simulink model "DFIPM_LinearModel"  (R2019b)
settings: Solver=FixedStepAuto  StartTime=0.0  StopTime=1  FixedStep=1e-7  RelTol=1e-3
values from neighbouring files (symbols this model uses):
  B = 0.00002    (= 2e-05)    [Parameter_Setting.m]
  duty_limit = 2/sqrt(3)    [Parameter_Setting.m]
  faif = 0.047    [Parameter_Setting.m]
  Iq_limit = 60    [Parameter_Setting.m]
  Jm = 0.00247*2    (= 0.00494)    [Parameter_Setting.m]
  Kawc = Kic/Kpc    (= 106.25)    [Parameter_Setting.m]
  Kic = Rs*wc    (= 106.814150222)    [Parameter_Setting.m]
  Kis = ws^2*Jm/KT    (= 276.628912008)    [Parameter_Setting.m]
  Kpc = Ld*wc    (= 1.00530964915)    [Parameter_Setting.m]
  Kps = yita*ws*2*Jm/KT    (= 3.1126989135)    [Parameter_Setting.m]
  Ld = 0.08e-3    (= 8e-05)    [Parameter_Setting.m]
  Lq = 0.28e-3    (= 0.00028)    [Parameter_Setting.m]
  p = 4    [Parameter_Setting.m]
  Rs = 8.5e-3    (= 0.0085)    [Parameter_Setting.m]
  Ts = 1/(50e3)    (= 2e-05)    [Parameter_Setting.m]
  Ts_spc = Ts    (= 2e-05)    [Parameter_Setting.m]
  VDC = 370    [Parameter_Setting.m]
undefined symbols (not defined in the file or in its folder): DiscIntNeverNeededParam
libraries: simulink x2, powerlib_meascontrol x1, powerlib x1
settings Model: Creator=Downstream  LastModifiedBy=Downstream
settings SolverCC: AlgebraicLoopSolver=LineSearch

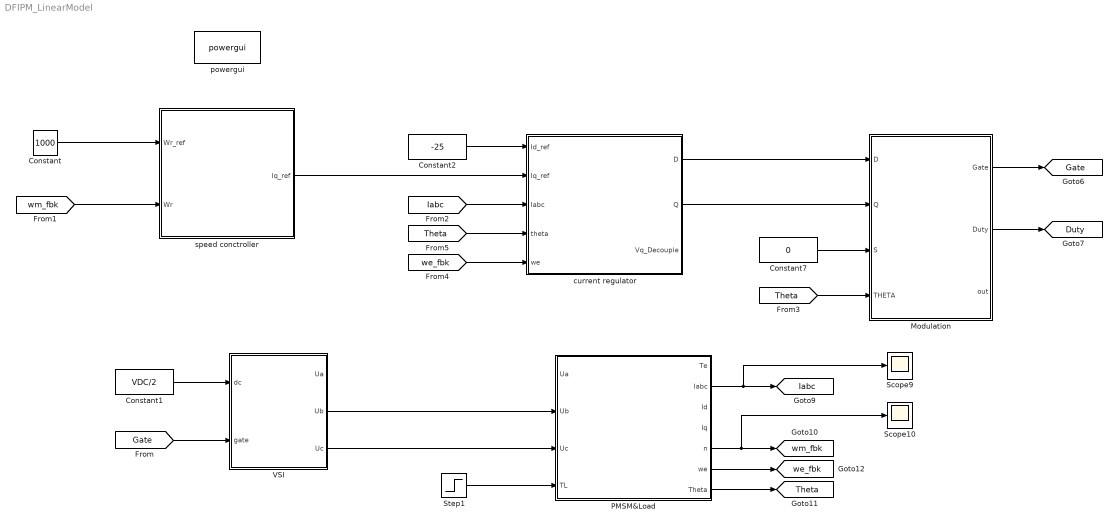
== system DFIPM_LinearModel ==
  Constant : Constant  Value=1000  OutDataTypeStr=Inherit: Inherit via back propagation  SampleTime=-1
  Constant1 : Constant  Value=VDC/2  SampleTime=-1
  Constant2 : Constant  Value=-25  SampleTime=-1
  Constant7 : Constant  Value=0  SampleTime=-1
  Modulation : Subsystem
  "PMSM&Load " : Subsystem
  Scope10 : Scope
  Scope9 : Scope
  Step1 : Step  Time=0.3  After=10
  VSI : Subsystem
  current regulator : Subsystem
  powergui : powerlib/powergui  Priority=1  SimulationMode=Discrete  SampleTime=1e-7  frequency=60  Iterations=50  frequencyindice=60  Pbase=100e6  ErrMax=1e-4  UnitsV=kV  UnitsW=MW  buscounter=0  FunctionMessages=off  echomessages=off  EnableUseOfTLC=off  CurrentSourceSwitches=off  DisableSnubberDevices=off  DisableRonSwitches=off  DisableVfSwitches=off  DisplayEquations=off  AutomaticDiscreteSolvers=off  SolverType=Tustin/Backward Euler (TBE)  Interpol=off  ExternalGateDelay=off  methode=off  Ts=100  x0status=blocks  SPID=on  SwTol=0  HookPort=off  NonlinearTolerance=1e-4  nMaxIteration=100  ContinueOnMaxIteration=off  RestoreLinks=warning  ResistiveCurrentMeasurement=off  Frange=[0:2:500]  Ylog=off  Xlog=on  ShowGrid=off  save=off  variable=ZData  structure=0  ZoomFFT=off  StartTime=0.0  cycles=1  DisplayStyle=1  fundamental=60  FreqAxis=off  MaxFrequency=1000  frequencyindicesteady=1  RmsSteady=1  display=off
      settings: SourceProductName=Simscape Electrical
  speed conctroller : Subsystem
  tag scope: Duty=global, Gate=global, Iabc=global, Theta=global, we_fbk=global, wm_fbk=global
  wires:
  Constant1/1 -> VSI/1(dc)
  VSI/2(Ub) -> "PMSM&Load "/2(Ub)
  VSI/3(Uc) -> "PMSM&Load "/3(Uc)
  [Gate] -> VSI/2(gate)
  speed conctroller/1(Iq_ref) -> current regulator/2(Iq_ref)
  [Iabc] -> current regulator/3(Iabc)
  [Theta] -> current regulator/4(theta)
  [we_fbk] -> current regulator/5(we)
  Modulation/1(Gate) -> [Gate]
  Constant/1 -> speed conctroller/1(Wr_ref)
  [Theta] -> Modulation/4(THETA)
  Constant7/1 -> Modulation/3(S)
  [wm_fbk] -> speed conctroller/2(Wr)
  Constant2/1 -> current regulator/1(Id_ref)
  Modulation/2(Duty) -> [Duty]
  current regulator/1(D) -> Modulation/1(D)
  current regulator/2(Q) -> Modulation/2(Q)
  "PMSM&Load "/2(Iabc) -> Scope9/1, [Iabc]
  "PMSM&Load "/5(n) -> Scope10/1, [wm_fbk]
  "PMSM&Load "/7(Theta) -> [Theta]
  "PMSM&Load "/6(we) -> [we_fbk]
  Step1/1 -> "PMSM&Load "/4(TL)

== system DFIPM_LinearModel/Modulation ==
  D : Inport
  Q : Inport  Port=2
  S : Inport  Port=3
  THETA : Inport  Port=4
  Mux : Mux  Inputs=3
  SVPWM1 : Subsystem
  Zero-Order Hold2 : ZeroOrderHold  SampleTime=Ts
  dq-abcde : Subsystem
  Gate : Outport  VectorParamsAs1DForOutWhenUnconnected=off
  Duty : Outport  Port=2  VectorParamsAs1DForOutWhenUnconnected=off
  out : Outport  Port=3  VectorParamsAs1DForOutWhenUnconnected=off
  wires:
  Q/1 -> dq-abcde/1(q1)
  D/1 -> dq-abcde/2(d1)
  S/1 -> dq-abcde/3(s)
  THETA/1 -> Zero-Order Hold2/1
  dq-abcde/2(B) -> Mux/2
  dq-abcde/3(C) -> Mux/3
  dq-abcde/1(A) -> Mux/1
  Mux/1 -> SVPWM1/1(Duty)
  SVPWM1/1(Gate) -> Gate/1
  Zero-Order Hold2/1 -> dq-abcde/4(Theta)
  SVPWM1/2(DutyCycle) -> Duty/1
  SVPWM1/3(out) -> out/1

== system DFIPM_LinearModel/PMSM&Load  ==
  Ua : Inport
  Ub : Inport  Port=2
  Uc : Inport  Port=3
  TL : Inport  Port=4
  PMSM : Subsystem
  Torque_Producer : Subsystem
  Te : Outport
  Iabc : Outport  Port=2
  Id : Outport  Port=3
  Iq : Outport  Port=4
  n : Outport  Port=5
  we : Outport  Port=6
  Theta : Outport  Port=7
  wires:
  PMSM/1(Te) -> Torque_Producer/2(sigma_Te), Te/1
  PMSM/3(Id) -> Id/1
  Ub/1 -> PMSM/2(Ub)
  Uc/1 -> PMSM/3(Uc)
  PMSM/2(Iabc) -> Iabc/1
  Ua/1 -> PMSM/1(Ua)
  PMSM/4(Iq) -> Iq/1
  TL/1 -> Torque_Producer/1(TL)
  Torque_Producer/1(n) -> n/1
  Torque_Producer/3(theta) -> Theta/1, PMSM/4(Theta)
  Torque_Producer/2(we) -> we/1

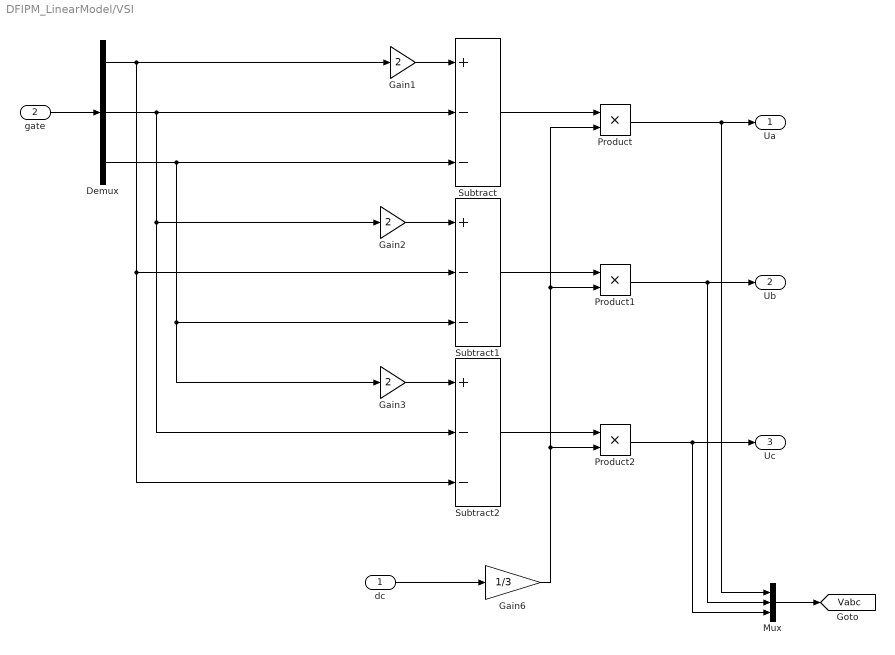
== system DFIPM_LinearModel/VSI ==
  dc : Inport
  gate : Inport  Port=2
  Demux : Demux  Outputs=3
  Gain1 : Gain  Gain=2
  Gain2 : Gain  Gain=2
  Gain3 : Gain  Gain=2
  Gain6 : Gain  Gain=1/3
  Mux : Mux  Inputs=3
  Product : Product  RndMeth=Zero
  Product1 : Product  RndMeth=Zero
  Product2 : Product  RndMeth=Zero
  Subtract : Sum  Inputs=+--
  Subtract1 : Sum  Inputs=+--
  Subtract2 : Sum  Inputs=+--
  Ua : Outport  VectorParamsAs1DForOutWhenUnconnected=off
  Ub : Outport  Port=2  VectorParamsAs1DForOutWhenUnconnected=off
  Uc : Outport  Port=3  VectorParamsAs1DForOutWhenUnconnected=off
  tag scope: Vabc=global
  wires:
  Demux/2 -> Subtract2/2, Gain2/1, Subtract/2
  Demux/3 -> Gain3/1, Subtract1/3, Subtract/3
  Product/1 -> Ua/1, Mux/1
  Product1/1 -> Mux/2, Ub/1
  Product2/1 -> Mux/3, Uc/1
  dc/1 -> Gain6/1
  Demux/1 -> Gain1/1, Subtract1/2, Subtract2/3
  Gain1/1 -> Subtract/1
  Subtract/1 -> Product/1
  Gain6/1 -> Product/2, Product1/2, Product2/2
  Gain2/1 -> Subtract1/1
  Subtract1/1 -> Product1/1
  Gain3/1 -> Subtract2/1
  Subtract2/1 -> Product2/1
  gate/1 -> Demux/1
  Mux/1 -> [Vabc]

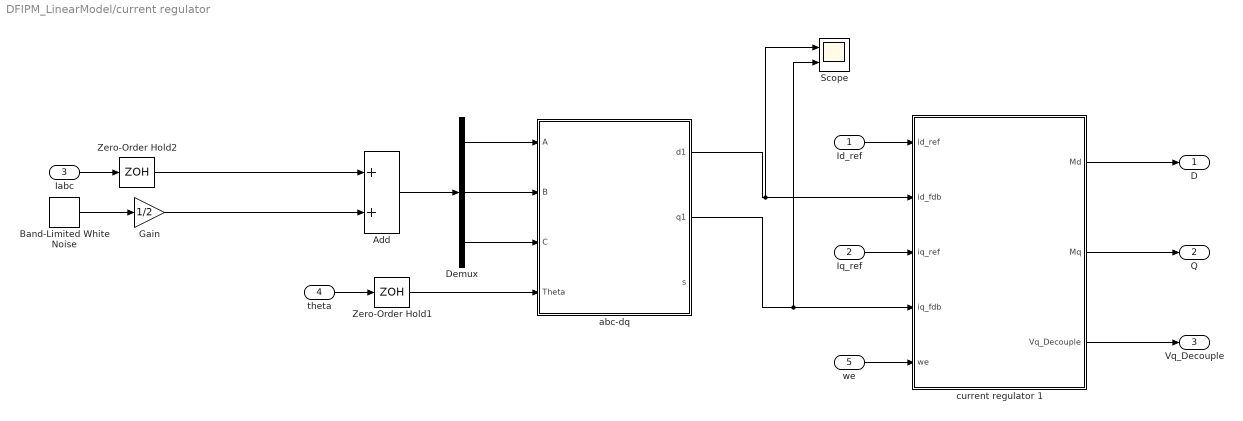
== system DFIPM_LinearModel/current regulator ==
  Id_ref : Inport
  Iq_ref : Inport  Port=2
  Iabc : Inport  Port=3
  theta : Inport  Port=4
  we : Inport  Port=5
  Add : Sum
  Band-Limited White Noise : simulink/Sources/Band-Limited White Noise  Cov=[0.003]  Ts=Ts  seed=[23341]
  Demux : Demux  Outputs=3
  Gain : Gain  Gain=1/2
  Scope : Scope  NumInputPorts=2
  Zero-Order Hold1 : ZeroOrderHold  SampleTime=Ts
  Zero-Order Hold2 : ZeroOrderHold  SampleTime=Ts
  abc-dq : Subsystem
  "current regulator 1 " : Subsystem
  D : Outport  VectorParamsAs1DForOutWhenUnconnected=off
  Q : Outport  Port=2  VectorParamsAs1DForOutWhenUnconnected=off
  Vq_Decouple : Outport  Port=3  VectorParamsAs1DForOutWhenUnconnected=off
  wires:
  Demux/3 -> abc-dq/3(C)
  Demux/1 -> abc-dq/1(A)
  theta/1 -> Zero-Order Hold1/1
  Iabc/1 -> Zero-Order Hold2/1
  Id_ref/1 -> "current regulator 1 "/1(id_ref)
  we/1 -> "current regulator 1 "/5(we)
  "current regulator 1 "/1(Md) -> D/1
  "current regulator 1 "/2(Mq) -> Q/1
  Demux/2 -> abc-dq/2(B)
  Zero-Order Hold1/1 -> abc-dq/4(Theta)
  "current regulator 1 "/3(Vq_Decouple) -> Vq_Decouple/1
  Iq_ref/1 -> "current regulator 1 "/3(iq_ref)
  Band-Limited White Noise/1 -> Gain/1
  Gain/1 -> Add/2
  Zero-Order Hold2/1 -> Add/1
  Add/1 -> Demux/1
  abc-dq/1(d1) -> "current regulator 1 "/2(id_fdb), Scope/1
  abc-dq/2(q1) -> Scope/2, "current regulator 1 "/4(iq_fdb)

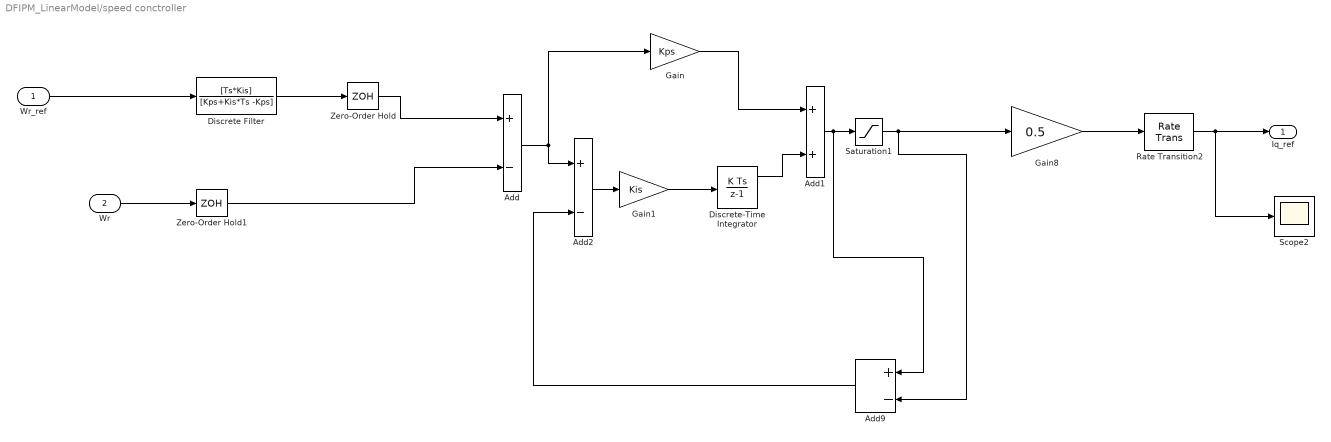
== system DFIPM_LinearModel/speed conctroller ==
  Wr_ref : Inport
  Wr : Inport  Port=2
  Add : Sum  Inputs=+-
  Add1 : Sum
  Add2 : Sum  Inputs=+-
  Add9 : Sum  Inputs=+-
  Discrete Filter : DiscreteFilter  Numerator=[Ts*Kis]  Denominator=[Kps+Kis*Ts -Kps]  SampleTime=Ts
  Discrete-Time Integrator : DiscreteIntegrator  gainval=1  SampleTime=Ts_spc  LimitOutput=on  UpperSaturationLimit=Iq_limit  LowerSaturationLimit=0  ShowSaturationPort=on  ICPrevOutput=DiscIntNeverNeededParam  ICPrevScaledInput=DiscIntNeverNeededParam
  Gain : Gain  Gain=Kps
  Gain1 : Gain  Gain=Kis
  Gain8 : Gain  Gain=0.5
  Rate Transition2 : RateTransition
  Saturation1 : Saturate  UpperLimit=Iq_limit  LowerLimit=-Iq_limit
  Scope2 : Scope
  Zero-Order Hold : ZeroOrderHold  SampleTime=Ts_spc
  Zero-Order Hold1 : ZeroOrderHold  SampleTime=Ts_spc
  Iq_ref : Outport  VectorParamsAs1DForOutWhenUnconnected=off
  wires:
  Gain/1 -> Add1/1
  Wr/1 -> Zero-Order Hold1/1
  Wr_ref/1 -> Discrete Filter/1
  Add1/1 -> Saturation1/1, Add9/1
  Saturation1/1 -> Gain8/1, Add9/2
  Rate Transition2/1 -> Scope2/1, Iq_ref/1
  Zero-Order Hold/1 -> Add/1
  Discrete Filter/1 -> Zero-Order Hold/1
  Discrete-Time Integrator/1 -> Add1/2
  Add/1 -> Add2/1, Gain/1
  Add2/1 -> Gain1/1
  Gain1/1 -> Discrete-Time Integrator/1
  Gain8/1 -> Rate Transition2/1
  Add9/1 -> Add2/2
  Zero-Order Hold1/1 -> Add/2

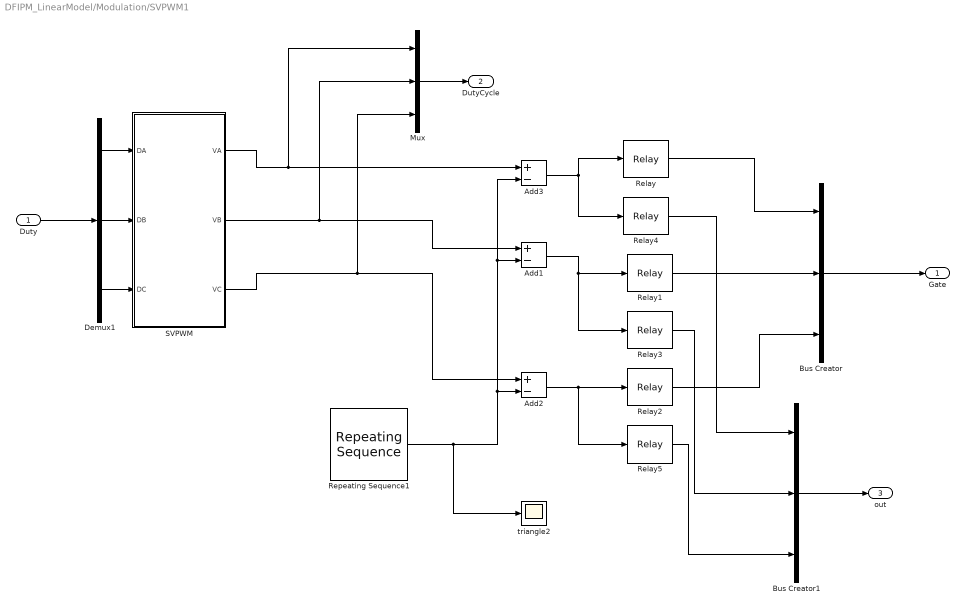
== system DFIPM_LinearModel/Modulation/SVPWM1 ==
  Duty : Inport
  Add1 : Sum  Inputs=+-
  Add2 : Sum  Inputs=+-
  Add3 : Sum  Inputs=+-
  Bus Creator : BusCreator  Inputs=3
  Bus Creator1 : BusCreator  Inputs=3
  Demux1 : Demux  Outputs=3
  Mux : Mux  Inputs=3
  Relay : Relay  OnSwitchValue=0  OffSwitchValue=0  OffOutputValue=-1
  Relay1 : Relay  OnSwitchValue=0  OffSwitchValue=0  OffOutputValue=-1
  Relay2 : Relay  OnSwitchValue=0  OffSwitchValue=0  OffOutputValue=-1
  Relay3 : Relay  OnSwitchValue=0  OffSwitchValue=0
  Relay4 : Relay  OnSwitchValue=0  OffSwitchValue=0
  Relay5 : Relay  OnSwitchValue=0  OffSwitchValue=0
  Repeating Sequence1 : simulink/Sources/Repeating Sequence  rep_seq_t=[0 Ts/2 Ts]  rep_seq_y=[-1 1 -1]
  SVPWM : Subsystem
  triangle2 : Scope
  Gate : Outport  VectorParamsAs1DForOutWhenUnconnected=off
  DutyCycle : Outport  Port=2  VectorParamsAs1DForOutWhenUnconnected=off
  out : Outport  Port=3  VectorParamsAs1DForOutWhenUnconnected=off
  wires:
  Duty/1 -> Demux1/1
  Add3/1 -> Relay/1, Relay4/1
  Add1/1 -> Relay3/1, Relay1/1
  Relay1/1 -> Bus Creator/2
  Add2/1 -> Relay5/1, Relay2/1
  Relay2/1 -> Bus Creator/3
  Relay/1 -> Bus Creator/1
  Bus Creator/1 -> Gate/1
  Demux1/1 -> SVPWM/1(DA)
  Demux1/2 -> SVPWM/2(DB)
  Demux1/3 -> SVPWM/3(DC)
  SVPWM/2(VB) -> Mux/2, Add1/1
  SVPWM/3(VC) -> Mux/3, Add2/1
  SVPWM/1(VA) -> Mux/1, Add3/1
  Mux/1 -> DutyCycle/1
  Repeating Sequence1/1 -> triangle2/1, Add1/2, Add3/2, Add2/2
  Relay4/1 -> Bus Creator1/1
  Relay3/1 -> Bus Creator1/2
  Relay5/1 -> Bus Creator1/3
  Bus Creator1/1 -> out/1

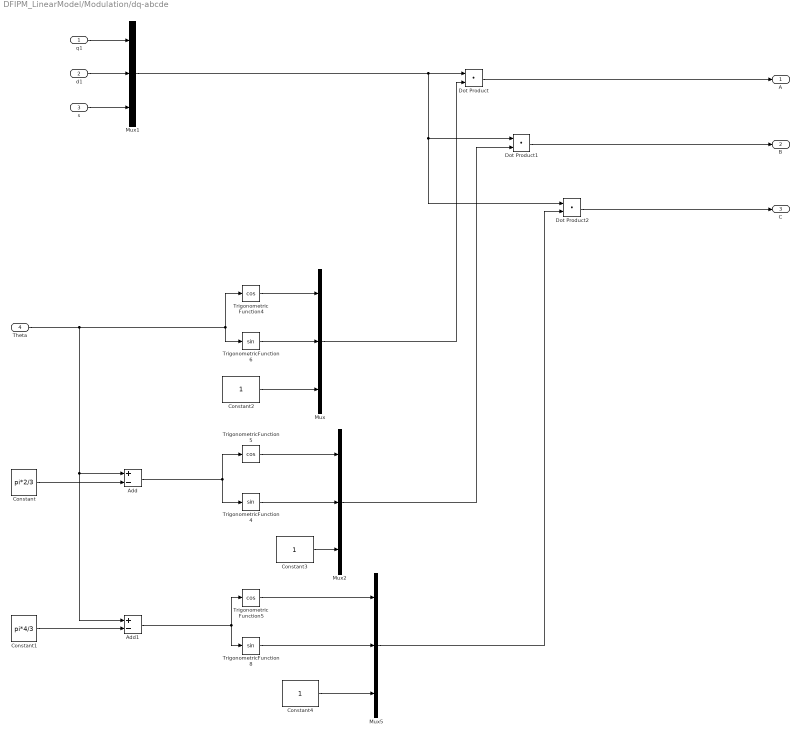
== system DFIPM_LinearModel/Modulation/dq-abcde ==
  q1 : Inport
  d1 : Inport  Port=2
  s : Inport  Port=3
  Theta : Inport  Port=4
  Add : Sum  Inputs=+-
  Add1 : Sum  Inputs=+-
  Constant : Constant  Value=pi*2/3
  Constant1 : Constant  Value=pi*4/3
  Constant2 : Constant
  Constant3 : Constant
  Constant4 : Constant
  Dot Product : DotProduct  InputSameDT=on  OutDataTypeStr=Inherit: Inherit via internal rule
  Dot Product1 : DotProduct  InputSameDT=on  OutDataTypeStr=Inherit: Inherit via internal rule
  Dot Product2 : DotProduct  InputSameDT=on  OutDataTypeStr=Inherit: Inherit via internal rule
  Mux{,1..2,5} (4 alike) : Mux  Inputs=3
  Trigonometric Function4 : Trigonometry  Operator=cos
  Trigonometric Function5 : Trigonometry  Operator=cos
  TrigonometricFunction4 : Trigonometry
  TrigonometricFunction5 : Trigonometry  Operator=cos
  TrigonometricFunction6 : Trigonometry
  TrigonometricFunction8 : Trigonometry
  A : Outport  VectorParamsAs1DForOutWhenUnconnected=off
  B : Outport  Port=2  VectorParamsAs1DForOutWhenUnconnected=off
  C : Outport  Port=3  VectorParamsAs1DForOutWhenUnconnected=off
  wires:
  Theta/1 -> Add/1, Add1/1, Trigonometric Function4/1, TrigonometricFunction6/1
  Constant/1 -> Add/2
  Constant1/1 -> Add1/2
  Add/1 -> TrigonometricFunction5/1, TrigonometricFunction4/1
  Add1/1 -> Trigonometric Function5/1, TrigonometricFunction8/1
  q1/1 -> Mux1/1
  d1/1 -> Mux1/2
  Mux/1 -> Dot Product/2
  Mux1/1 -> Dot Product/1, Dot Product1/1, Dot Product2/1
  Mux2/1 -> Dot Product1/2
  Mux5/1 -> Dot Product2/2
  Trigonometric Function4/1 -> Mux/1
  TrigonometricFunction6/1 -> Mux/2
  TrigonometricFunction5/1 -> Mux2/1
  TrigonometricFunction4/1 -> Mux2/2
  TrigonometricFunction8/1 -> Mux5/2
  Trigonometric Function5/1 -> Mux5/1
  ? -> ?
  Dot Product/1 -> A/1
  Dot Product1/1 -> B/1
  Dot Product2/1 -> C/1
  Constant3/1 -> Mux2/3
  Constant4/1 -> Mux5/3
  Constant2/1 -> Mux/3
  s/1 -> Mux1/3

== system DFIPM_LinearModel/PMSM&Load /PMSM ==
  Ua : Inport
  Ub : Inport  Port=2
  Uc : Inport  Port=3
  Theta : Inport  Port=4
  Mux : Mux  Inputs=3
  Voltage to Current : Subsystem
  abc-dq : Subsystem
  dq-abc : Subsystem
  Te : Outport  VectorParamsAs1DForOutWhenUnconnected=off
  Iabc : Outport  Port=2  VectorParamsAs1DForOutWhenUnconnected=off
  Id : Outport  Port=3  VectorParamsAs1DForOutWhenUnconnected=off
  Iq : Outport  Port=4  VectorParamsAs1DForOutWhenUnconnected=off
  wires:
  abc-dq/2(q1) -> Voltage to Current/2(Uq)
  Mux/1 -> Iabc/1
  dq-abc/3(C) -> Mux/3
  Voltage to Current/3(Te) -> Te/1
  dq-abc/2(B) -> Mux/2
  Voltage to Current/1(Id) -> Id/1, dq-abc/1(d1)
  Ua/1 -> abc-dq/1(A)
  Uc/1 -> abc-dq/3(C)
  Voltage to Current/2(Iq) -> Iq/1, dq-abc/2(q1)
  Ub/1 -> abc-dq/2(B)
  dq-abc/1(A) -> Mux/1
  abc-dq/1(01) -> Voltage to Current/1(Ud)
  Theta/1 -> dq-abc/4(Theta), abc-dq/4(Theta)

== system DFIPM_LinearModel/PMSM&Load /Torque_Producer ==
  TL : Inport
  sigma_Te : Inport  Port=2
  Add4 : Sum  Inputs=+--
  Gain11 : Gain  Gain=B
  Gain12 : Gain  Gain=1/Jm
  Gain13 : Gain  Gain=p
  Gain14 : Gain  Gain=30/pi
  Integrator2 : Integrator
  Integrator3 : Integrator
  n : Outport  VectorParamsAs1DForOutWhenUnconnected=off
  we : Outport  Port=2  VectorParamsAs1DForOutWhenUnconnected=off
  theta : Outport  Port=3  VectorParamsAs1DForOutWhenUnconnected=off
  tag scope: w=global
  wires:
  sigma_Te/1 -> Add4/1
  TL/1 -> Add4/2
  [w] -> Gain11/1
  Gain11/1 -> Add4/3
  Add4/1 -> Gain12/1
  Gain12/1 -> Integrator2/1
  Integrator2/1 -> Gain14/1, [w]
  Integrator3/1 -> theta/1
  [w] -> Gain13/1
  Gain13/1 -> we/1, Integrator3/1
  Gain14/1 -> n/1

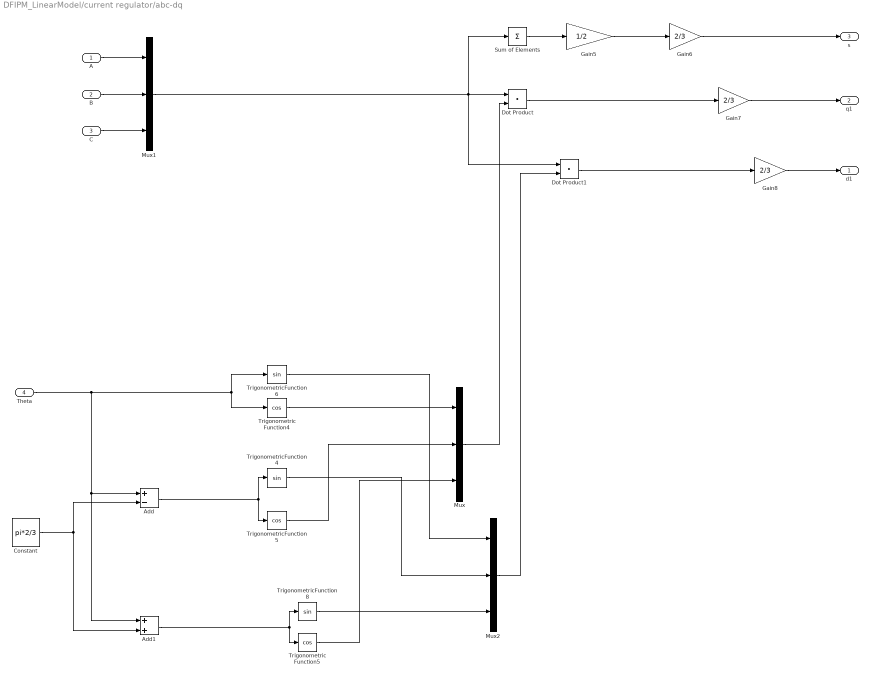
== system DFIPM_LinearModel/current regulator/abc-dq ==
  A : Inport
  B : Inport  Port=2
  C : Inport  Port=3
  Theta : Inport  Port=4
  Add : Sum  Inputs=+-
  Add1 : Sum
  Constant : Constant  Value=pi*2/3
  Dot Product : DotProduct  InputSameDT=on  OutDataTypeStr=Inherit: Inherit via internal rule
  Dot Product1 : DotProduct  InputSameDT=on  OutDataTypeStr=Inherit: Inherit via internal rule
  Gain5 : Gain  Gain=1/2
  Gain6 : Gain  Gain=2/3
  Gain7 : Gain  Gain=2/3
  Gain8 : Gain  Gain=2/3
  Mux : Mux  Inputs=3
  Mux1 : Mux  Inputs=3
  Mux2 : Mux  Inputs=3
  Sum of Elements : Sum  Inputs=+
  Trigonometric Function4 : Trigonometry  Operator=cos
  Trigonometric Function5 : Trigonometry  Operator=cos
  TrigonometricFunction4 : Trigonometry
  TrigonometricFunction5 : Trigonometry  Operator=cos
  TrigonometricFunction6 : Trigonometry
  TrigonometricFunction8 : Trigonometry
  d1 : Outport  VectorParamsAs1DForOutWhenUnconnected=off
  q1 : Outport  Port=2  VectorParamsAs1DForOutWhenUnconnected=off
  s : Outport  Port=3  VectorParamsAs1DForOutWhenUnconnected=off
  wires:
  Theta/1 -> Add/1, Add1/1, TrigonometricFunction6/1, Trigonometric Function4/1
  Constant/1 -> Add/2, Add1/2
  Add/1 -> TrigonometricFunction4/1, TrigonometricFunction5/1
  Add1/1 -> TrigonometricFunction8/1, Trigonometric Function5/1
  A/1 -> Mux1/1
  B/1 -> Mux1/2
  C/1 -> Mux1/3
  Mux/1 -> Dot Product/2
  Mux1/1 -> Dot Product/1, Sum of Elements/1, Dot Product1/1
  Dot Product/1 -> Gain7/1
  Mux2/1 -> Dot Product1/2
  Dot Product1/1 -> Gain8/1
  Sum of Elements/1 -> Gain5/1
  Gain5/1 -> Gain6/1
  Gain6/1 -> s/1
  Gain7/1 -> q1/1
  Gain8/1 -> d1/1
  Trigonometric Function4/1 -> Mux/1
  TrigonometricFunction5/1 -> Mux/2
  Trigonometric Function5/1 -> Mux/3
  TrigonometricFunction6/1 -> Mux2/1
  TrigonometricFunction4/1 -> Mux2/2
  TrigonometricFunction8/1 -> Mux2/3

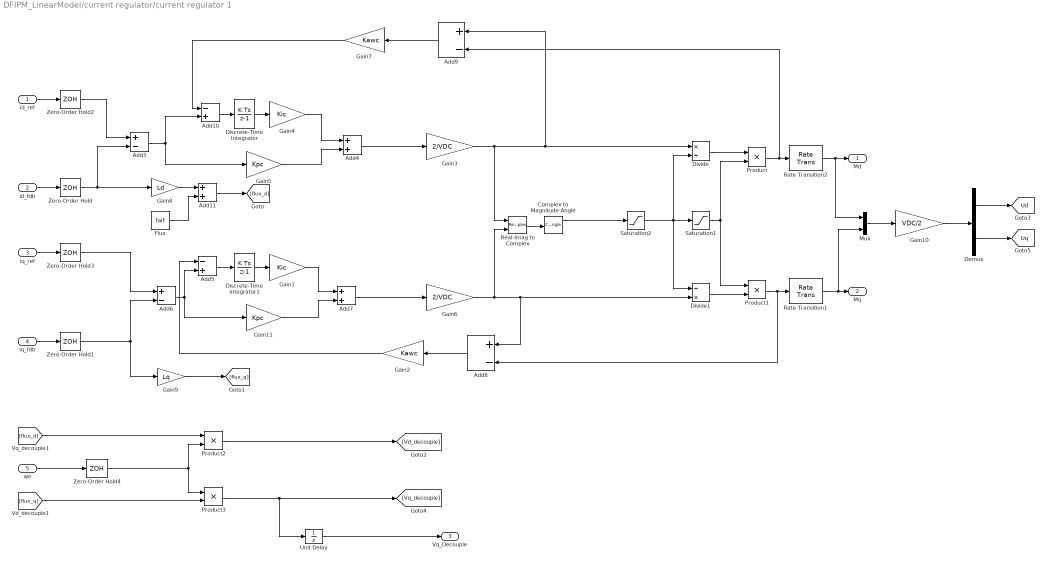
== system DFIPM_LinearModel/current regulator/current regulator 1  ==
  id_ref : Inport
  id_fdb : Inport  Port=2
  iq_ref : Inport  Port=3
  iq_fdb : Inport  Port=4
  we : Inport  Port=5
  Add10 : Sum  Inputs=-+
  Add11 : Sum
  Add{3,6,8..9} (4 alike) : Sum  Inputs=+-
  Add4 : Sum
  Add5 : Sum  Inputs=-+
  Add7 : Sum
  Complex to Magnitude-Angle : ComplexToMagnitudeAngle
  Demux : Demux  Outputs=2
  Discrete-Time Integrator : DiscreteIntegrator  SampleTime=Ts  ICPrevOutput=DiscIntNeverNeededParam  ICPrevScaledInput=DiscIntNeverNeededParam
  Discrete-Time Integrator1 : DiscreteIntegrator  SampleTime=Ts  ICPrevOutput=DiscIntNeverNeededParam  ICPrevScaledInput=DiscIntNeverNeededParam
  Divide : Product  Inputs=*/
  Divide1 : Product  Inputs=/*
  Flux : Constant  Value=faif  SampleTime=-1
  Gain1 : Gain  Gain=Kic
  Gain10 : Gain  Gain=VDC/2
  Gain11 : Gain  Gain=Kpc
  Gain2 : Gain  Gain=Kawc
  Gain3 : Gain  Gain=2/VDC
  Gain4 : Gain  Gain=Kic
  Gain5 : Gain  Gain=Kpc
  Gain6 : Gain  Gain=2/VDC
  Gain7 : Gain  Gain=Kawc
  Gain8 : Gain  Gain=Ld
  Gain9 : Gain  Gain=Lq
  Mux : Mux  Inputs=2
  Product{,1..3} (4 alike) : Product
  Rate Transition1 : RateTransition
  Rate Transition2 : RateTransition
  Real-Imag to Complex : RealImagToComplex
  Saturation1 : Saturate  UpperLimit=duty_limit  LowerLimit=0
  Saturation2 : Saturate  UpperLimit=800  LowerLimit=1e-9
  Unit Delay : UnitDelay  SampleTime=-1  HasFrameUpgradeWarning=on
  Zero-Order Hold{,1..4} (5 alike) : ZeroOrderHold  SampleTime=Ts
  Md : Outport  VectorParamsAs1DForOutWhenUnconnected=off
  Mq : Outport  Port=2  VectorParamsAs1DForOutWhenUnconnected=off
  Vq_Decouple : Outport  Port=3  VectorParamsAs1DForOutWhenUnconnected=off
  tag scope: Ud=global, Uq=global
  wires:
  id_fdb/1 -> Zero-Order Hold/1
  id_ref/1 -> Zero-Order Hold2/1
  Discrete-Time Integrator/1 -> Gain4/1
  Gain4/1 -> Add4/1
  Gain5/1 -> Add4/2
  Zero-Order Hold2/1 -> Add3/1
  Rate Transition2/1 -> Mux/1, Md/1
  Zero-Order Hold/1 -> Gain8/1, Add3/2
  Add3/1 -> Gain5/1, Add10/2
  iq_fdb/1 -> Zero-Order Hold1/1
  iq_ref/1 -> Zero-Order Hold3/1
  Discrete-Time Integrator1/1 -> Gain1/1
  Add6/1 -> Gain11/1, Add5/2
  Gain1/1 -> Add7/1
  Gain11/1 -> Add7/2
  Zero-Order Hold3/1 -> Add6/1
  Zero-Order Hold1/1 -> Gain9/1, Add6/2
  Add5/1 -> Discrete-Time Integrator1/1
  Add4/1 -> Gain3/1
  Add7/1 -> Gain6/1
  Gain3/1 -> Real-Imag to Complex/1, Add9/1, Divide/1
  Real-Imag to Complex/1 -> Complex to Magnitude-Angle/1
  Complex to Magnitude-Angle/1 -> Saturation2/1
  Divide/1 -> Product/1
  Saturation1/1 -> Product/2, Product1/1
  Product/1 -> Add9/2, Rate Transition2/1
  Rate Transition1/1 -> Mux/2, Mq/1
  Gain6/1 -> Real-Imag to Complex/2, Add8/1, Divide1/2
  Product1/1 -> Add8/2, Rate Transition1/1
  Divide1/1 -> Product1/2
  Add8/1 -> Gain2/1
  Gain8/1 -> Add11/1
  Flux/1 -> Add11/2
  Add11/1 -> [flux_d]
  Gain9/1 -> [flux_q]
  [flux_d] -> Product2/1
  we/1 -> Zero-Order Hold4/1
  [flux_q] -> Product3/2
  Product2/1 -> [Vd_decouple]
  Product3/1 -> Unit Delay/1, [Vq_decouple]
  Zero-Order Hold4/1 -> Product3/1, Product2/2
  Gain2/1 -> Add5/1
  Add9/1 -> Gain7/1
  Add10/1 -> Discrete-Time Integrator/1
  Gain7/1 -> Add10/1
  Unit Delay/1 -> Vq_Decouple/1
  Mux/1 -> Gain10/1
  Gain10/1 -> Demux/1
  Demux/1 -> [Ud]
  Demux/2 -> [Uq]
  Saturation2/1 -> Divide1/1, Divide/2, Saturation1/1

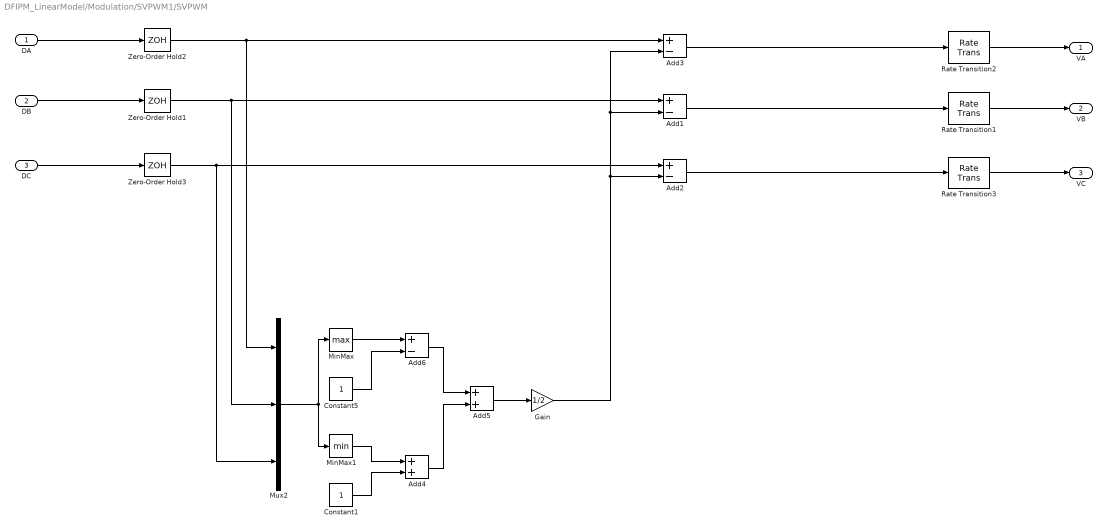
== system DFIPM_LinearModel/Modulation/SVPWM1/SVPWM ==
  DA : Inport
  DB : Inport  Port=2
  DC : Inport  Port=3
  Add{1..3,6} (4 alike) : Sum  Inputs=+-
  Add4 : Sum
  Add5 : Sum
  Constant1 : Constant
  Constant5 : Constant
  Gain : Gain  Gain=1/2
  MinMax : MinMax  Function=max
  MinMax1 : MinMax
  Mux2 : Mux  Inputs=3
  Rate Transition1 : RateTransition  OutPortSampleTime=Ts
  Rate Transition2 : RateTransition  OutPortSampleTime=Ts
  Rate Transition3 : RateTransition  OutPortSampleTime=Ts
  Zero-Order Hold1 : ZeroOrderHold  SampleTime=Ts
  Zero-Order Hold2 : ZeroOrderHold  SampleTime=Ts
  Zero-Order Hold3 : ZeroOrderHold  SampleTime=Ts
  VA : Outport  VectorParamsAs1DForOutWhenUnconnected=off
  VB : Outport  Port=2  VectorParamsAs1DForOutWhenUnconnected=off
  VC : Outport  Port=3  VectorParamsAs1DForOutWhenUnconnected=off
  wires:
  DA/1 -> Zero-Order Hold2/1
  DB/1 -> Zero-Order Hold1/1
  DC/1 -> Zero-Order Hold3/1
  Add2/1 -> Rate Transition3/1
  Add1/1 -> Rate Transition1/1
  Add3/1 -> Rate Transition2/1
  Mux2/1 -> MinMax/1, MinMax1/1
  MinMax/1 -> Add6/1
  Constant5/1 -> Add6/2
  Rate Transition2/1 -> VA/1
  Rate Transition1/1 -> VB/1
  Rate Transition3/1 -> VC/1
  MinMax1/1 -> Add4/1
  Constant1/1 -> Add4/2
  Add6/1 -> Add5/1
  Add4/1 -> Add5/2
  Add5/1 -> Gain/1
  Gain/1 -> Add3/2, Add1/2, Add2/2
  Zero-Order Hold2/1 -> Add3/1, Mux2/1
  Zero-Order Hold1/1 -> Add1/1, Mux2/2
  Zero-Order Hold3/1 -> Add2/1, Mux2/3

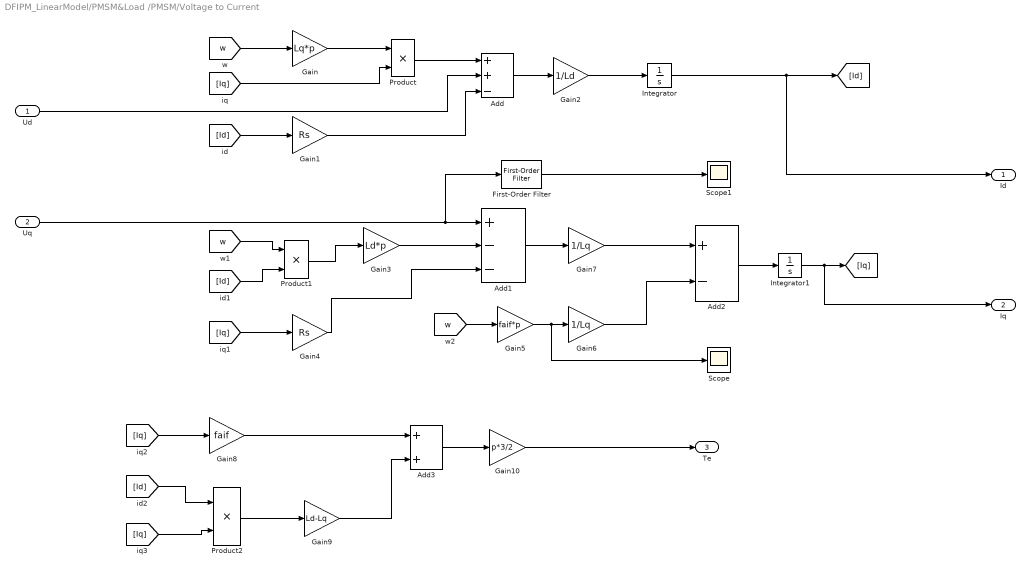
== system DFIPM_LinearModel/PMSM&Load /PMSM/Voltage to Current ==
  Ud : Inport
  Uq : Inport  Port=2
  Add : Sum  Inputs=++-
  Add1 : Sum  Inputs=+--
  Add2 : Sum  Inputs=+-
  Add3 : Sum
  First-Order Filter : powerlib_meascontrol/Filters/First-Order Filter  FilterType=Lowpass  Tc=10e-3  Ts=0  Initialize=off  Vac_Init=[0, 0, 60]  Vdc_Init=0  PlotResponse=off  FreqRange="[0,  200,  1]"
      settings: SourceProductName=Simscape Electrical
  Gain : Gain  Gain=Lq*p
  Gain1 : Gain  Gain=Rs
  Gain10 : Gain  Gain=p*3/2
  Gain2 : Gain  Gain=1/Ld
  Gain3 : Gain  Gain=Ld*p
  Gain4 : Gain  Gain=Rs
  Gain5 : Gain  Gain=faif*p
  Gain6 : Gain  Gain=1/Lq
  Gain7 : Gain  Gain=1/Lq
  Gain8 : Gain  Gain=faif
  Gain9 : Gain  Gain=Ld-Lq
  Integrator : Integrator
  Integrator1 : Integrator
  Product : Product
  Product1 : Product
  Product2 : Product
  Scope : Scope
  Scope1 : Scope
  Id : Outport  VectorParamsAs1DForOutWhenUnconnected=off
  Iq : Outport  Port=2  VectorParamsAs1DForOutWhenUnconnected=off
  Te : Outport  Port=3  VectorParamsAs1DForOutWhenUnconnected=off
  wires:
  Gain/1 -> Product/1
  [Iq] -> Product/2
  [w] -> Gain/1
  Ud/1 -> Add/2
  Product/1 -> Add/1
  [Id] -> Gain1/1
  Gain1/1 -> Add/3
  Add/1 -> Gain2/1
  Uq/1 -> First-Order Filter/1, Add1/1
  [w] -> Product1/1
  [Id] -> Product1/2
  Product1/1 -> Gain3/1
  Gain3/1 -> Add1/2
  [Iq] -> Gain4/1
  Gain4/1 -> Add1/3
  [w] -> Gain5/1
  Gain5/1 -> Scope/1, Gain6/1
  Add1/1 -> Gain7/1
  Gain7/1 -> Add2/1
  Gain6/1 -> Add2/2
  Gain2/1 -> Integrator/1
  Integrator/1 -> Id/1, [Id]
  Add2/1 -> Integrator1/1
  Integrator1/1 -> Iq/1, [Iq]
  [Iq] -> Gain8/1
  Gain8/1 -> Add3/1
  [Id] -> Product2/1
  [Iq] -> Product2/2
  Product2/1 -> Gain9/1
  Gain9/1 -> Add3/2
  Add3/1 -> Gain10/1
  Gain10/1 -> Te/1
  First-Order Filter/1 -> Scope1/1

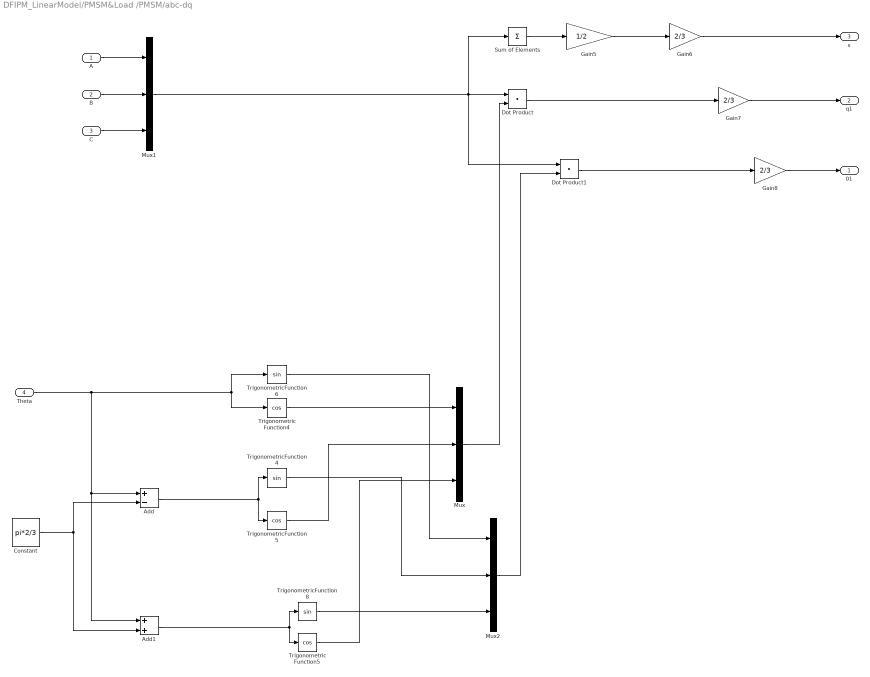
== system DFIPM_LinearModel/PMSM&Load /PMSM/abc-dq ==
  A : Inport
  B : Inport  Port=2
  C : Inport  Port=3
  Theta : Inport  Port=4
  Add : Sum  Inputs=+-
  Add1 : Sum
  Constant : Constant  Value=pi*2/3  SampleTime=-1
  Dot Product : DotProduct  InputSameDT=on  OutDataTypeStr=Inherit: Inherit via internal rule
  Dot Product1 : DotProduct  InputSameDT=on  OutDataTypeStr=Inherit: Inherit via internal rule
  Gain5 : Gain  Gain=1/2
  Gain6 : Gain  Gain=2/3
  Gain7 : Gain  Gain=2/3
  Gain8 : Gain  Gain=2/3
  Mux : Mux  Inputs=3
  Mux1 : Mux  Inputs=3
  Mux2 : Mux  Inputs=3
  Sum of Elements : Sum  Inputs=+
  Trigonometric Function4 : Trigonometry  Operator=cos
  Trigonometric Function5 : Trigonometry  Operator=cos
  TrigonometricFunction4 : Trigonometry
  TrigonometricFunction5 : Trigonometry  Operator=cos
  TrigonometricFunction6 : Trigonometry
  TrigonometricFunction8 : Trigonometry
  01 : Outport  VectorParamsAs1DForOutWhenUnconnected=off
  q1 : Outport  Port=2  VectorParamsAs1DForOutWhenUnconnected=off
  s : Outport  Port=3  VectorParamsAs1DForOutWhenUnconnected=off
  wires:
  Theta/1 -> Add/1, Add1/1, TrigonometricFunction6/1, Trigonometric Function4/1
  Constant/1 -> Add/2, Add1/2
  Add/1 -> TrigonometricFunction4/1, TrigonometricFunction5/1
  Add1/1 -> TrigonometricFunction8/1, Trigonometric Function5/1
  A/1 -> Mux1/1
  B/1 -> Mux1/2
  C/1 -> Mux1/3
  Mux/1 -> Dot Product/2
  Mux1/1 -> Dot Product/1, Sum of Elements/1, Dot Product1/1
  Dot Product/1 -> Gain7/1
  Mux2/1 -> Dot Product1/2
  Dot Product1/1 -> Gain8/1
  Sum of Elements/1 -> Gain5/1
  Gain5/1 -> Gain6/1
  Gain6/1 -> s/1
  Gain7/1 -> q1/1
  Gain8/1 -> 01/1
  Trigonometric Function4/1 -> Mux/1
  TrigonometricFunction5/1 -> Mux/2
  Trigonometric Function5/1 -> Mux/3
  TrigonometricFunction6/1 -> Mux2/1
  TrigonometricFunction4/1 -> Mux2/2
  TrigonometricFunction8/1 -> Mux2/3

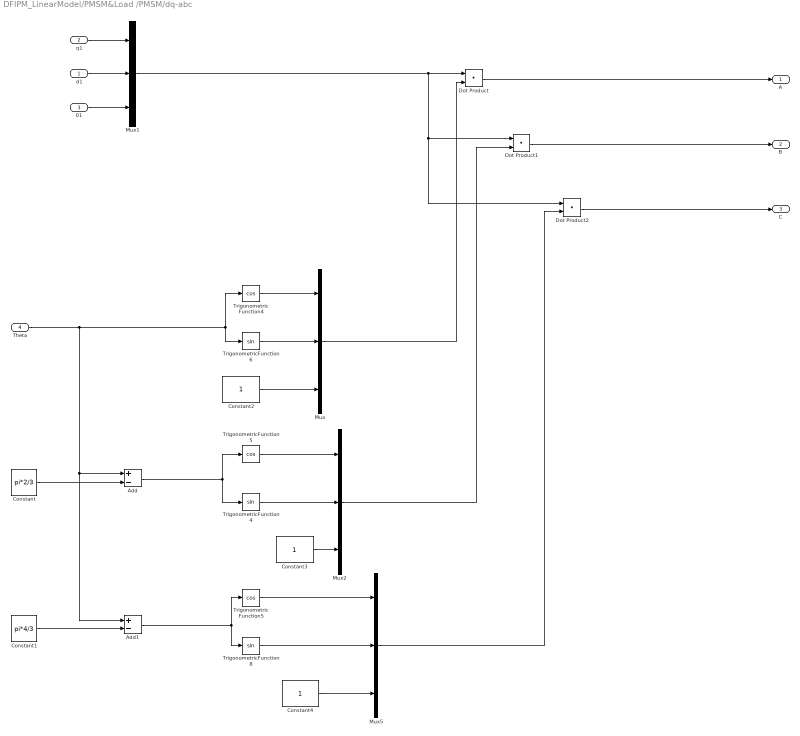
== system DFIPM_LinearModel/PMSM&Load /PMSM/dq-abc ==
  d1 : Inport
  q1 : Inport  Port=2
  01 : Inport  Port=3
  Theta : Inport  Port=4
  Add : Sum  Inputs=+-
  Add1 : Sum  Inputs=+-
  Constant : Constant  Value=pi*2/3
  Constant1 : Constant  Value=pi*4/3
  Constant2 : Constant
  Constant3 : Constant
  Constant4 : Constant
  Dot Product : DotProduct  InputSameDT=on  OutDataTypeStr=Inherit: Inherit via internal rule
  Dot Product1 : DotProduct  InputSameDT=on  OutDataTypeStr=Inherit: Inherit via internal rule
  Dot Product2 : DotProduct  InputSameDT=on  OutDataTypeStr=Inherit: Inherit via internal rule
  Mux{,1..2,5} (4 alike) : Mux  Inputs=3
  Trigonometric Function4 : Trigonometry  Operator=cos
  Trigonometric Function5 : Trigonometry  Operator=cos
  TrigonometricFunction4 : Trigonometry
  TrigonometricFunction5 : Trigonometry  Operator=cos
  TrigonometricFunction6 : Trigonometry
  TrigonometricFunction8 : Trigonometry
  A : Outport  VectorParamsAs1DForOutWhenUnconnected=off
  B : Outport  Port=2  VectorParamsAs1DForOutWhenUnconnected=off
  C : Outport  Port=3  VectorParamsAs1DForOutWhenUnconnected=off
  wires:
  Theta/1 -> Add/1, Add1/1, Trigonometric Function4/1, TrigonometricFunction6/1
  Constant/1 -> Add/2
  Constant1/1 -> Add1/2
  Add/1 -> TrigonometricFunction5/1, TrigonometricFunction4/1
  Add1/1 -> Trigonometric Function5/1, TrigonometricFunction8/1
  q1/1 -> Mux1/1
  d1/1 -> Mux1/2
  Mux/1 -> Dot Product/2
  Mux1/1 -> Dot Product/1, Dot Product1/1, Dot Product2/1
  Mux2/1 -> Dot Product1/2
  Mux5/1 -> Dot Product2/2
  Trigonometric Function4/1 -> Mux/1
  TrigonometricFunction6/1 -> Mux/2
  TrigonometricFunction5/1 -> Mux2/1
  TrigonometricFunction4/1 -> Mux2/2
  TrigonometricFunction8/1 -> Mux5/2
  Trigonometric Function5/1 -> Mux5/1
  ? -> ?
  Dot Product/1 -> A/1
  Dot Product1/1 -> B/1
  Dot Product2/1 -> C/1
  Constant3/1 -> Mux2/3
  Constant4/1 -> Mux5/3
  Constant2/1 -> Mux/3
  01/1 -> Mux1/3
